simulink model "complexModel"  (R2025a)
settings: Solver=VariableStepAuto  StartTime=0.0  StopTime=10.0  RelTol=1e-3
libraries: simulink x1
settings Model: Creator=willager  LastModifiedBy=willager

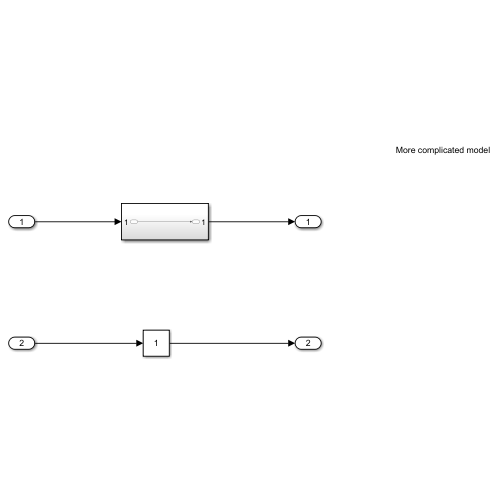
[thumbnail: Simulink's stored preview of the top-level diagram]
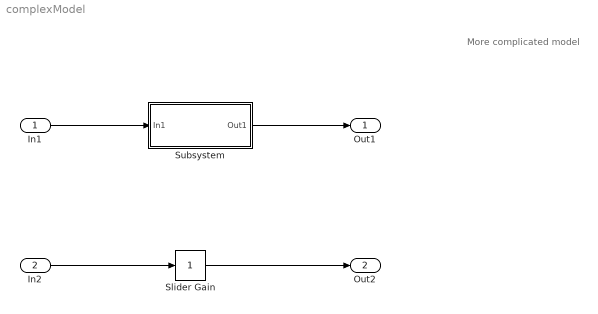
== system complexModel ==
  note: More complicated model
  In1 : Inport
  In2 : Inport  Port=2
  Slider Gain : simulink/Math Operations/Slider Gain  gain=1  low=0  high=2
  Subsystem : Subsystem
  Out1 : Outport
  Out2 : Outport  Port=2
  wires:
  Subsystem/1(Out1) -> Out1/1
  In1/1 -> Subsystem/1(In1)
  In2/1 -> Slider Gain/1
  Slider Gain/1 -> Out2/1

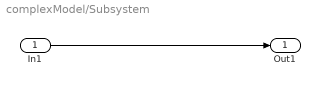
== system complexModel/Subsystem ==
  In1 : Inport
  Out1 : Outport
  wires:
  In1/1 -> Out1/1
